simulink model "problem3"  (R2020a)
settings: Solver=VariableStepAuto  StartTime=0.0  StopTime=10.0  RelTol=1e-3
model workspace (MAT data in the model file):
  Ki = Simulink.Parameter
  Ki.Value = 50
  Ki.DataType = 'auto'
  Ki.Dimensions = [1 1]
  Kp = Simulink.Parameter
  Kp.Value = 800
  Kp.DataType = 'auto'
  Kp.Dimensions = [1 1]
  ki = Simulink.Parameter
  ki.Value = 50
  ki.DataType = 'auto'
  ki.Dimensions = [1 1]
  kp = Simulink.Parameter
  kp.Value = 800
  kp.DataType = 'auto'
  kp.Dimensions = [1 1]
settings Model: OrderedModelArguments=off  Creator=Riyansh  LastModifiedBy=Riyansh

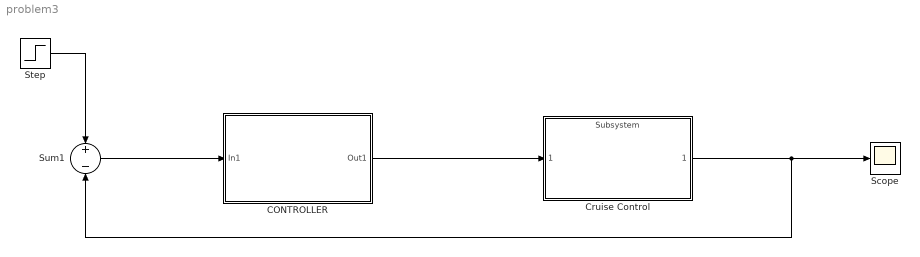
== system problem3 ==
  CONTROLLER : Subsystem
  Cruise Control : ModelReference  ModelNameDialog=Subsystem  ModelReferenceVersion=1.6
  Scope : Scope
  Step : Step  After=u  SampleTime=0
  Sum1 : Sum  Inputs=+-
  wires:
  Step/1 -> Sum1/1
  Sum1/1 -> CONTROLLER/1(In1)
  CONTROLLER/1(Out1) -> Cruise Control/1
  Cruise Control/1 -> Sum1/2, Scope/1

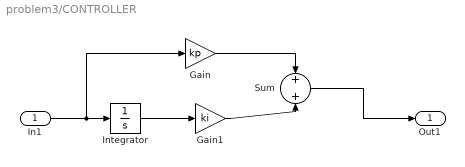
== system problem3/CONTROLLER ==
  In1 : Inport
  Gain : Gain  Gain=kp
  Gain1 : Gain  Gain=ki
  Integrator : Integrator
  Sum : Sum
  Out1 : Outport
  wires:
  Sum/1 -> Out1/1
  In1/1 -> Gain/1, Integrator/1
  Integrator/1 -> Gain1/1
  Gain1/1 -> Sum/2
  Gain/1 -> Sum/1
